simulink model "Basic_1"  (R2020a)
settings: Solver=VariableStepAuto  StartTime=0.0  StopTime=20.0  RelTol=1e-3
model workspace (MAT data in the model file):
  F10 = [0  0; 0.015  28.22; 0.077  26.082; 0.201  24.934; 0.31  22.806; 0.464  20.183; 0.573  17.886; 0.789  16.075; 1.068  13.946; 1.393  12.63; 1.718  11.155; 2.166  9.844; 2.677  9.515; 3.311  9.187; 3.683  8.859; 3.791  9.679; 4.101  9.679; 4.658  9.515; 5.168  9.023; 5.725  9.023; 6.112  8.531; 6.329  8.859; 6.499  7.546; 6.685  5.742; 6.778  4.921; 6.917  2.625; 7.025  1.312; 7.13  0; 7.5  0]
libraries: simulink x2, shared3dof x1, simulink_extras x1
settings Model: PacingRate=0.100000  Creator=jdoos  LastModifiedBy=jdoos

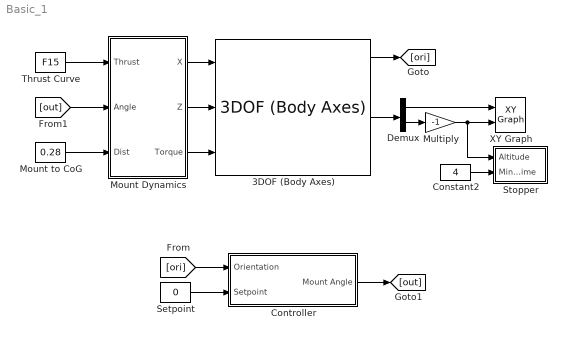
== system Basic_1 ==
  3DOF (Body Axes) : shared3dof/3DOF (Body Axes)  units=Metric (MKS)  mtype=Fixed  v_ini=0  theta_ini=0  alpha_ini=0  pos_ini=[0 0]  q_ini=0  mass=0.543  mass_e=0.5  mass_f=3.0  Iyy=0.048  Iyy_e=0.5  Iyy_f=3.0  g_in=Internal  g=9.81  vre_flag=on  abi_flag=off  aMode=0  vel_statename=''  theta_statename=''  pos_statename=''  q_statename=''  mass_statename=''
      settings: SourceProductBaseCode=AE,PW,MT,VE,VP
  Constant2 : Constant  Value=4
  Controller : Subsystem
  Demux : Demux  Outputs=2
  Mount Dynamics : Subsystem
  Mount to CoG : Constant  Value=0.28
  Multiply : Gain  Gain=-1
  Setpoint : Constant  Value=0
  Stopper : Subsystem
  Thrust Curve : FromWorkspace  VariableName=F15
  XY Graph : simulink/Sinks/XY Graph  xmin=-50  xmax=50  ymin=0  ymax=300  st=-1
  wires:
  Mount Dynamics/1(X) -> 3DOF (Body Axes)/1
  Mount Dynamics/2(Z) -> 3DOF (Body Axes)/2
  Mount Dynamics/3(Torque) -> 3DOF (Body Axes)/3
  [out] -> Mount Dynamics/2(Angle)
  Mount to CoG/1 -> Mount Dynamics/3(Dist)
  3DOF (Body Axes)/4 -> Demux/1
  Demux/1 -> XY Graph/1
  Demux/2 -> Multiply/1
  Multiply/1 -> XY Graph/2, Stopper/1(Altitude)
  Constant2/1 -> Stopper/2(Min Time)
  Thrust Curve/1 -> Mount Dynamics/1(Thrust)
  3DOF (Body Axes)/1 -> [ori]
  [ori] -> Controller/1(Orientation)
  Controller/1(Mount Angle) -> [out]
  Setpoint/1 -> Controller/2(Setpoint)

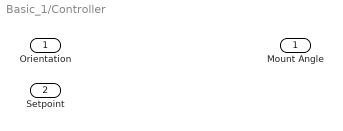
== system Basic_1/Controller ==
  Orientation : Inport
  Setpoint : Inport  Port=2
  Mount Angle : Outport

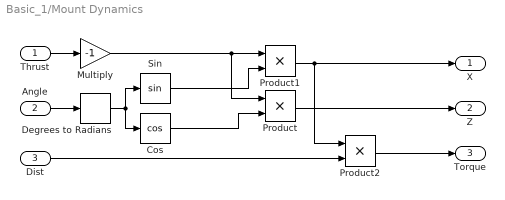
== system Basic_1/Mount Dynamics ==
  Thrust : Inport
  Angle : Inport  Port=2
  Dist : Inport  Port=3
  Cos : Trigonometry  Operator=cos
  Degrees to Radians : simulink_extras/Transformations/Degrees to Radians
  Multiply : Gain  Gain=-1
  Product : Product
  Product1 : Product
  Product2 : Product
  Sin : Trigonometry
  X : Outport
  Z : Outport  Port=2
  Torque : Outport  Port=3
  wires:
  Thrust/1 -> Multiply/1
  Sin/1 -> Product1/2
  Cos/1 -> Product/2
  Dist/1 -> Product2/2
  Product2/1 -> Torque/1
  Product1/1 -> Product2/1, X/1
  Product/1 -> Z/1
  Multiply/1 -> Product/1, Product1/1
  Angle/1 -> Degrees to Radians/1
  Degrees to Radians/1 -> Cos/1, Sin/1

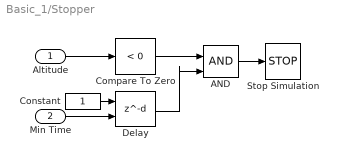
== system Basic_1/Stopper ==
  Altitude : Inport
  Min Time : Inport  Port=2
  AND : Logic  IconShape=distinctive  AllPortsSameDT=off  OutDataTypeStr=boolean
  Compare To Zero : simulink/Logic and Bit Operations/Compare To Zero  relop=<  OutDataTypeStr=boolean
  Constant : Constant
  Delay : Delay  DelayLengthSource=Input port
      settings: InputPortMap=u0,p1
  Stop Simulation : Stop
  wires:
  AND/1 -> Stop Simulation/1
  Compare To Zero/1 -> AND/1
  Altitude/1 -> Compare To Zero/1
  Delay/1 -> AND/2
  Min Time/1 -> Delay/2
  Constant/1 -> Delay/1
